simulink model "test1s"  (R2021a)
settings: Solver=VariableStepAuto  StartTime=0.0  StopTime=10.0  RelTol=1e-3
values from neighbouring files (symbols this model uses):
  y = Q*a0    [L1_4_sec_fft.m]    (also in L1_5_sec_dst.m; L1_5sec_dct.m; L1_dct_6_sec.m; L1_dst_4_sec.m)
settings Model: Creator=yadu1  LastModifiedBy=yadu1

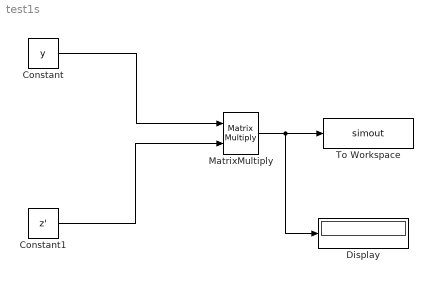
== system test1s ==
  Constant : Constant  Value=y
  Constant1 : Constant  Value=z'  VectorParams1D=off
  Display : Display
  MatrixMultiply : Product  Multiplication=Matrix(*)
  To Workspace : ToWorkspace  VariableName=simout  SaveFormat=Timeseries  SampleTime=-1
  wires:
  Constant/1 -> MatrixMultiply/1
  Constant1/1 -> MatrixMultiply/2
  MatrixMultiply/1 -> Display/1, To Workspace/1
